simulink model "EV_assigment2"  (R2022a)
settings: Solver=VariableStepAuto  StartTime=0.0  StopTime=10800  RelTol=1e-3
libraries: spsCurrentMeasurementLib x141, spsSeriesRLCBranchLib x141, spsVoltageMeasurementLib x141, spsControlledVoltageSourceLib x140, spspowerguiLib x1
(part 8 of 15)

== system EV_assigment2/series/Subsystem15/Subsystem ==
  SOC : Inport
  Battery temp : Inport  Port=2
  2-D Lookup Table : Lookup_n-D  BreakpointsForDimension1=[0 0.10 0.20 0.30 0.40 0.50 0.60 0.70 0.80 0.90 1]  BreakpointsForDimension2=[293.15 313.15]  Table=[3.50 3.51;3.56 3.56; 3.60 3.62;3.64 3.66;3.67 3.69;3.71 3.72;3.79 3.81;3.88 3.89;3.97 3.99;4.08 4.08;4.19 4.19]  InternalRulePriority=Speed  RndMeth=Simplest
      settings: InputPortMap=u0,u1
  2-D Lookup Table1 : Lookup_n-D  BreakpointsForDimension1=[0 0.10 0.20 0.30 0.40 0.50 0.60 0.70 0.80 0.90 1]  BreakpointsForDimension2=[293.15 313.15]  Table=[0.011448 0.009001;0.011038 0.008966;0.011281 0.009126;0.011236 0.00911;0.010959 0.008957;0.010714 0.008797;0.010698 0.008913;0.010712 0.009052;0.010917 0.009044;0.011304 0.008899;0.01160 0.008902]  InternalRulePriority=Speed  RndMeth=Simplest
      settings: InputPortMap=u0,u1
  2-D Lookup Table2 : Lookup_n-D  BreakpointsForDimension1=[0 0.10 0.20 0.30 0.40 0.50 0.60 0.70 0.80 0.90 1]  BreakpointsForDimension2=[293.15 313.15]  Table=[0.010342 0;0.006732 0.10;0.005116 0.20;0.004345 0.30;0.003883 0.40;0.003423 0.50;0.003346 0.60;0.003322 0.70;0.00332 0.80;0.003289 0.90;0.002811 1]  InternalRulePriority=Speed  RndMeth=Simplest
      settings: InputPortMap=u0,u1
  2-D Lookup Table3 : Lookup_n-D  BreakpointsForDimension1=[0 0.10 0.20 0.30 0.40 0.50 0.60 0.70 0.8 0.9 1]  BreakpointsForDimension2=[293.15 313.15]  Table=[2287.7 11897;6122 24515;18460 42098;20975 44453;15254 33098;10440 24492;13903 32975;16694 40007;15784 35937;12165 26430;9118 24795]  InternalRulePriority=Speed  RndMeth=Simplest
      settings: InputPortMap=u0,u1
  Em : Outport
  R0 : Outport  Port=2
  R1 : Outport  Port=3
  C1 : Outport  Port=4
  wires:
  Battery temp/1 -> 2-D Lookup Table3/2, 2-D Lookup Table2/2, 2-D Lookup Table1/2, 2-D Lookup Table/2
  2-D Lookup Table3/1 -> C1/1
  2-D Lookup Table/1 -> Em/1
  SOC/1 -> 2-D Lookup Table3/1, 2-D Lookup Table2/1, 2-D Lookup Table1/1, 2-D Lookup Table/1
  2-D Lookup Table2/1 -> R1/1
  2-D Lookup Table1/1 -> R0/1

== system EV_assigment2/series/Subsystem15/Subsystem1 ==
  Battery Current : Inport
  InitCap(Ah) : Inport  Port=2
  Temp(K) : Inport  Port=3
  Capacity : Lookup_n-D  NumberOfTableDimensions=1  BreakpointsForDimension1=[283.15 313.15]  Table=[28 28]  InternalRulePriority=Speed  RndMeth=Simplest
  Charge accumilator : Integrator  InitialConditionSource=external  UpperSaturationLimit=1  LowerSaturationLimit=0
  Convert to Ah : Gain  Gain=-1/3600
  Divide : Product  Inputs=*/
  LoadAh : Outport
  SOC : Outport  Port=2
  wires:
  Charge accumilator/1 -> Divide/1, LoadAh/1
  Divide/1 -> SOC/1
  Temp(K)/1 -> Capacity/1
  Capacity/1 -> Divide/2
  Battery Current/1 -> Convert to Ah/1
  Convert to Ah/1 -> Charge accumilator/1
  InitCap(Ah)/1 -> Charge accumilator/2

== system EV_assigment2/series/Subsystem16/Subsystem ==
  SOC : Inport
  Battery temp : Inport  Port=2
  2-D Lookup Table : Lookup_n-D  BreakpointsForDimension1=[0 0.10 0.20 0.30 0.40 0.50 0.60 0.70 0.80 0.90 1]  BreakpointsForDimension2=[293.15 313.15]  Table=[3.50 3.51;3.56 3.56; 3.60 3.62;3.64 3.66;3.67 3.69;3.71 3.72;3.79 3.81;3.88 3.89;3.97 3.99;4.08 4.08;4.19 4.19]  InternalRulePriority=Speed  RndMeth=Simplest
      settings: InputPortMap=u0,u1
  2-D Lookup Table1 : Lookup_n-D  BreakpointsForDimension1=[0 0.10 0.20 0.30 0.40 0.50 0.60 0.70 0.80 0.90 1]  BreakpointsForDimension2=[293.15 313.15]  Table=[0.011448 0.009001;0.011038 0.008966;0.011281 0.009126;0.011236 0.00911;0.010959 0.008957;0.010714 0.008797;0.010698 0.008913;0.010712 0.009052;0.010917 0.009044;0.011304 0.008899;0.01160 0.008902]  InternalRulePriority=Speed  RndMeth=Simplest
      settings: InputPortMap=u0,u1
  2-D Lookup Table2 : Lookup_n-D  BreakpointsForDimension1=[0 0.10 0.20 0.30 0.40 0.50 0.60 0.70 0.80 0.90 1]  BreakpointsForDimension2=[293.15 313.15]  Table=[0.010342 0;0.006732 0.10;0.005116 0.20;0.004345 0.30;0.003883 0.40;0.003423 0.50;0.003346 0.60;0.003322 0.70;0.00332 0.80;0.003289 0.90;0.002811 1]  InternalRulePriority=Speed  RndMeth=Simplest
      settings: InputPortMap=u0,u1
  2-D Lookup Table3 : Lookup_n-D  BreakpointsForDimension1=[0 0.10 0.20 0.30 0.40 0.50 0.60 0.70 0.8 0.9 1]  BreakpointsForDimension2=[293.15 313.15]  Table=[2287.7 11897;6122 24515;18460 42098;20975 44453;15254 33098;10440 24492;13903 32975;16694 40007;15784 35937;12165 26430;9118 24795]  InternalRulePriority=Speed  RndMeth=Simplest
      settings: InputPortMap=u0,u1
  Em : Outport
  R0 : Outport  Port=2
  R1 : Outport  Port=3
  C1 : Outport  Port=4
  wires:
  Battery temp/1 -> 2-D Lookup Table3/2, 2-D Lookup Table2/2, 2-D Lookup Table1/2, 2-D Lookup Table/2
  2-D Lookup Table3/1 -> C1/1
  2-D Lookup Table/1 -> Em/1
  SOC/1 -> 2-D Lookup Table3/1, 2-D Lookup Table2/1, 2-D Lookup Table1/1, 2-D Lookup Table/1
  2-D Lookup Table2/1 -> R1/1
  2-D Lookup Table1/1 -> R0/1

== system EV_assigment2/series/Subsystem16/Subsystem1 ==
  Battery Current : Inport
  InitCap(Ah) : Inport  Port=2
  Temp(K) : Inport  Port=3
  Capacity : Lookup_n-D  NumberOfTableDimensions=1  BreakpointsForDimension1=[283.15 313.15]  Table=[28 28]  InternalRulePriority=Speed  RndMeth=Simplest
  Charge accumilator : Integrator  InitialConditionSource=external  UpperSaturationLimit=1  LowerSaturationLimit=0
  Convert to Ah : Gain  Gain=-1/3600
  Divide : Product  Inputs=*/
  LoadAh : Outport
  SOC : Outport  Port=2
  wires:
  Charge accumilator/1 -> Divide/1, LoadAh/1
  Divide/1 -> SOC/1
  Temp(K)/1 -> Capacity/1
  Capacity/1 -> Divide/2
  Battery Current/1 -> Convert to Ah/1
  Convert to Ah/1 -> Charge accumilator/1
  InitCap(Ah)/1 -> Charge accumilator/2

== system EV_assigment2/series/Subsystem17/Subsystem ==
  SOC : Inport
  Battery temp : Inport  Port=2
  2-D Lookup Table : Lookup_n-D  BreakpointsForDimension1=[0 0.10 0.20 0.30 0.40 0.50 0.60 0.70 0.80 0.90 1]  BreakpointsForDimension2=[293.15 313.15]  Table=[3.50 3.51;3.56 3.56; 3.60 3.62;3.64 3.66;3.67 3.69;3.71 3.72;3.79 3.81;3.88 3.89;3.97 3.99;4.08 4.08;4.19 4.19]  InternalRulePriority=Speed  RndMeth=Simplest
      settings: InputPortMap=u0,u1
  2-D Lookup Table1 : Lookup_n-D  BreakpointsForDimension1=[0 0.10 0.20 0.30 0.40 0.50 0.60 0.70 0.80 0.90 1]  BreakpointsForDimension2=[293.15 313.15]  Table=[0.011448 0.009001;0.011038 0.008966;0.011281 0.009126;0.011236 0.00911;0.010959 0.008957;0.010714 0.008797;0.010698 0.008913;0.010712 0.009052;0.010917 0.009044;0.011304 0.008899;0.01160 0.008902]  InternalRulePriority=Speed  RndMeth=Simplest
      settings: InputPortMap=u0,u1
  2-D Lookup Table2 : Lookup_n-D  BreakpointsForDimension1=[0 0.10 0.20 0.30 0.40 0.50 0.60 0.70 0.80 0.90 1]  BreakpointsForDimension2=[293.15 313.15]  Table=[0.010342 0;0.006732 0.10;0.005116 0.20;0.004345 0.30;0.003883 0.40;0.003423 0.50;0.003346 0.60;0.003322 0.70;0.00332 0.80;0.003289 0.90;0.002811 1]  InternalRulePriority=Speed  RndMeth=Simplest
      settings: InputPortMap=u0,u1
  2-D Lookup Table3 : Lookup_n-D  BreakpointsForDimension1=[0 0.10 0.20 0.30 0.40 0.50 0.60 0.70 0.8 0.9 1]  BreakpointsForDimension2=[293.15 313.15]  Table=[2287.7 11897;6122 24515;18460 42098;20975 44453;15254 33098;10440 24492;13903 32975;16694 40007;15784 35937;12165 26430;9118 24795]  InternalRulePriority=Speed  RndMeth=Simplest
      settings: InputPortMap=u0,u1
  Em : Outport
  R0 : Outport  Port=2
  R1 : Outport  Port=3
  C1 : Outport  Port=4
  wires:
  Battery temp/1 -> 2-D Lookup Table3/2, 2-D Lookup Table2/2, 2-D Lookup Table1/2, 2-D Lookup Table/2
  2-D Lookup Table3/1 -> C1/1
  2-D Lookup Table/1 -> Em/1
  SOC/1 -> 2-D Lookup Table3/1, 2-D Lookup Table2/1, 2-D Lookup Table1/1, 2-D Lookup Table/1
  2-D Lookup Table2/1 -> R1/1
  2-D Lookup Table1/1 -> R0/1

== system EV_assigment2/series/Subsystem17/Subsystem1 ==
  Battery Current : Inport
  InitCap(Ah) : Inport  Port=2
  Temp(K) : Inport  Port=3
  Capacity : Lookup_n-D  NumberOfTableDimensions=1  BreakpointsForDimension1=[283.15 313.15]  Table=[28 28]  InternalRulePriority=Speed  RndMeth=Simplest
  Charge accumilator : Integrator  InitialConditionSource=external  UpperSaturationLimit=1  LowerSaturationLimit=0
  Convert to Ah : Gain  Gain=-1/3600
  Divide : Product  Inputs=*/
  LoadAh : Outport
  SOC : Outport  Port=2
  wires:
  Charge accumilator/1 -> Divide/1, LoadAh/1
  Divide/1 -> SOC/1
  Temp(K)/1 -> Capacity/1
  Capacity/1 -> Divide/2
  Battery Current/1 -> Convert to Ah/1
  Convert to Ah/1 -> Charge accumilator/1
  InitCap(Ah)/1 -> Charge accumilator/2

== system EV_assigment2/series/Subsystem18/Subsystem ==
  SOC : Inport
  Battery temp : Inport  Port=2
  2-D Lookup Table : Lookup_n-D  BreakpointsForDimension1=[0 0.10 0.20 0.30 0.40 0.50 0.60 0.70 0.80 0.90 1]  BreakpointsForDimension2=[293.15 313.15]  Table=[3.50 3.51;3.56 3.56; 3.60 3.62;3.64 3.66;3.67 3.69;3.71 3.72;3.79 3.81;3.88 3.89;3.97 3.99;4.08 4.08;4.19 4.19]  InternalRulePriority=Speed  RndMeth=Simplest
      settings: InputPortMap=u0,u1
  2-D Lookup Table1 : Lookup_n-D  BreakpointsForDimension1=[0 0.10 0.20 0.30 0.40 0.50 0.60 0.70 0.80 0.90 1]  BreakpointsForDimension2=[293.15 313.15]  Table=[0.011448 0.009001;0.011038 0.008966;0.011281 0.009126;0.011236 0.00911;0.010959 0.008957;0.010714 0.008797;0.010698 0.008913;0.010712 0.009052;0.010917 0.009044;0.011304 0.008899;0.01160 0.008902]  InternalRulePriority=Speed  RndMeth=Simplest
      settings: InputPortMap=u0,u1
  2-D Lookup Table2 : Lookup_n-D  BreakpointsForDimension1=[0 0.10 0.20 0.30 0.40 0.50 0.60 0.70 0.80 0.90 1]  BreakpointsForDimension2=[293.15 313.15]  Table=[0.010342 0;0.006732 0.10;0.005116 0.20;0.004345 0.30;0.003883 0.40;0.003423 0.50;0.003346 0.60;0.003322 0.70;0.00332 0.80;0.003289 0.90;0.002811 1]  InternalRulePriority=Speed  RndMeth=Simplest
      settings: InputPortMap=u0,u1
  2-D Lookup Table3 : Lookup_n-D  BreakpointsForDimension1=[0 0.10 0.20 0.30 0.40 0.50 0.60 0.70 0.8 0.9 1]  BreakpointsForDimension2=[293.15 313.15]  Table=[2287.7 11897;6122 24515;18460 42098;20975 44453;15254 33098;10440 24492;13903 32975;16694 40007;15784 35937;12165 26430;9118 24795]  InternalRulePriority=Speed  RndMeth=Simplest
      settings: InputPortMap=u0,u1
  Em : Outport
  R0 : Outport  Port=2
  R1 : Outport  Port=3
  C1 : Outport  Port=4
  wires:
  Battery temp/1 -> 2-D Lookup Table3/2, 2-D Lookup Table2/2, 2-D Lookup Table1/2, 2-D Lookup Table/2
  2-D Lookup Table3/1 -> C1/1
  2-D Lookup Table/1 -> Em/1
  SOC/1 -> 2-D Lookup Table3/1, 2-D Lookup Table2/1, 2-D Lookup Table1/1, 2-D Lookup Table/1
  2-D Lookup Table2/1 -> R1/1
  2-D Lookup Table1/1 -> R0/1

== system EV_assigment2/series/Subsystem18/Subsystem1 ==
  Battery Current : Inport
  InitCap(Ah) : Inport  Port=2
  Temp(K) : Inport  Port=3
  Capacity : Lookup_n-D  NumberOfTableDimensions=1  BreakpointsForDimension1=[283.15 313.15]  Table=[28 28]  InternalRulePriority=Speed  RndMeth=Simplest
  Charge accumilator : Integrator  InitialConditionSource=external  UpperSaturationLimit=1  LowerSaturationLimit=0
  Convert to Ah : Gain  Gain=-1/3600
  Divide : Product  Inputs=*/
  LoadAh : Outport
  SOC : Outport  Port=2
  wires:
  Charge accumilator/1 -> Divide/1, LoadAh/1
  Divide/1 -> SOC/1
  Temp(K)/1 -> Capacity/1
  Capacity/1 -> Divide/2
  Battery Current/1 -> Convert to Ah/1
  Convert to Ah/1 -> Charge accumilator/1
  InitCap(Ah)/1 -> Charge accumilator/2

== system EV_assigment2/series/Subsystem19/Subsystem ==
  SOC : Inport
  Battery temp : Inport  Port=2
  2-D Lookup Table : Lookup_n-D  BreakpointsForDimension1=[0 0.10 0.20 0.30 0.40 0.50 0.60 0.70 0.80 0.90 1]  BreakpointsForDimension2=[293.15 313.15]  Table=[3.50 3.51;3.56 3.56; 3.60 3.62;3.64 3.66;3.67 3.69;3.71 3.72;3.79 3.81;3.88 3.89;3.97 3.99;4.08 4.08;4.19 4.19]  InternalRulePriority=Speed  RndMeth=Simplest
      settings: InputPortMap=u0,u1
  2-D Lookup Table1 : Lookup_n-D  BreakpointsForDimension1=[0 0.10 0.20 0.30 0.40 0.50 0.60 0.70 0.80 0.90 1]  BreakpointsForDimension2=[293.15 313.15]  Table=[0.011448 0.009001;0.011038 0.008966;0.011281 0.009126;0.011236 0.00911;0.010959 0.008957;0.010714 0.008797;0.010698 0.008913;0.010712 0.009052;0.010917 0.009044;0.011304 0.008899;0.01160 0.008902]  InternalRulePriority=Speed  RndMeth=Simplest
      settings: InputPortMap=u0,u1
  2-D Lookup Table2 : Lookup_n-D  BreakpointsForDimension1=[0 0.10 0.20 0.30 0.40 0.50 0.60 0.70 0.80 0.90 1]  BreakpointsForDimension2=[293.15 313.15]  Table=[0.010342 0;0.006732 0.10;0.005116 0.20;0.004345 0.30;0.003883 0.40;0.003423 0.50;0.003346 0.60;0.003322 0.70;0.00332 0.80;0.003289 0.90;0.002811 1]  InternalRulePriority=Speed  RndMeth=Simplest
      settings: InputPortMap=u0,u1
  2-D Lookup Table3 : Lookup_n-D  BreakpointsForDimension1=[0 0.10 0.20 0.30 0.40 0.50 0.60 0.70 0.8 0.9 1]  BreakpointsForDimension2=[293.15 313.15]  Table=[2287.7 11897;6122 24515;18460 42098;20975 44453;15254 33098;10440 24492;13903 32975;16694 40007;15784 35937;12165 26430;9118 24795]  InternalRulePriority=Speed  RndMeth=Simplest
      settings: InputPortMap=u0,u1
  Em : Outport
  R0 : Outport  Port=2
  R1 : Outport  Port=3
  C1 : Outport  Port=4
  wires:
  Battery temp/1 -> 2-D Lookup Table3/2, 2-D Lookup Table2/2, 2-D Lookup Table1/2, 2-D Lookup Table/2
  2-D Lookup Table3/1 -> C1/1
  2-D Lookup Table/1 -> Em/1
  SOC/1 -> 2-D Lookup Table3/1, 2-D Lookup Table2/1, 2-D Lookup Table1/1, 2-D Lookup Table/1
  2-D Lookup Table2/1 -> R1/1
  2-D Lookup Table1/1 -> R0/1

== system EV_assigment2/series/Subsystem19/Subsystem1 ==
  Battery Current : Inport
  InitCap(Ah) : Inport  Port=2
  Temp(K) : Inport  Port=3
  Capacity : Lookup_n-D  NumberOfTableDimensions=1  BreakpointsForDimension1=[283.15 313.15]  Table=[28 28]  InternalRulePriority=Speed  RndMeth=Simplest
  Charge accumilator : Integrator  InitialConditionSource=external  UpperSaturationLimit=1  LowerSaturationLimit=0
  Convert to Ah : Gain  Gain=-1/3600
  Divide : Product  Inputs=*/
  LoadAh : Outport
  SOC : Outport  Port=2
  wires:
  Charge accumilator/1 -> Divide/1, LoadAh/1
  Divide/1 -> SOC/1
  Temp(K)/1 -> Capacity/1
  Capacity/1 -> Divide/2
  Battery Current/1 -> Convert to Ah/1
  Convert to Ah/1 -> Charge accumilator/1
  InitCap(Ah)/1 -> Charge accumilator/2

== system EV_assigment2/series/Subsystem2/Subsystem ==
  SOC : Inport
  Battery temp : Inport  Port=2
  2-D Lookup Table : Lookup_n-D  BreakpointsForDimension1=[0 0.10 0.20 0.30 0.40 0.50 0.60 0.70 0.80 0.90 1]  BreakpointsForDimension2=[293.15 313.15]  Table=[3.50 3.51;3.56 3.56; 3.60 3.62;3.64 3.66;3.67 3.69;3.71 3.72;3.79 3.81;3.88 3.89;3.97 3.99;4.08 4.08;4.19 4.19]  InternalRulePriority=Speed  RndMeth=Simplest
      settings: InputPortMap=u0,u1
  2-D Lookup Table1 : Lookup_n-D  BreakpointsForDimension1=[0 0.10 0.20 0.30 0.40 0.50 0.60 0.70 0.80 0.90 1]  BreakpointsForDimension2=[293.15 313.15]  Table=[0.011448 0.009001;0.011038 0.008966;0.011281 0.009126;0.011236 0.00911;0.010959 0.008957;0.010714 0.008797;0.010698 0.008913;0.010712 0.009052;0.010917 0.009044;0.011304 0.008899;0.01160 0.008902]  InternalRulePriority=Speed  RndMeth=Simplest
      settings: InputPortMap=u0,u1
  2-D Lookup Table2 : Lookup_n-D  BreakpointsForDimension1=[0 0.10 0.20 0.30 0.40 0.50 0.60 0.70 0.80 0.90 1]  BreakpointsForDimension2=[293.15 313.15]  Table=[0.010342 0;0.006732 0.10;0.005116 0.20;0.004345 0.30;0.003883 0.40;0.003423 0.50;0.003346 0.60;0.003322 0.70;0.00332 0.80;0.003289 0.90;0.002811 1]  InternalRulePriority=Speed  RndMeth=Simplest
      settings: InputPortMap=u0,u1
  2-D Lookup Table3 : Lookup_n-D  BreakpointsForDimension1=[0 0.10 0.20 0.30 0.40 0.50 0.60 0.70 0.8 0.9 1]  BreakpointsForDimension2=[293.15 313.15]  Table=[2287.7 11897;6122 24515;18460 42098;20975 44453;15254 33098;10440 24492;13903 32975;16694 40007;15784 35937;12165 26430;9118 24795]  InternalRulePriority=Speed  RndMeth=Simplest
      settings: InputPortMap=u0,u1
  Em : Outport
  R0 : Outport  Port=2
  R1 : Outport  Port=3
  C1 : Outport  Port=4
  wires:
  Battery temp/1 -> 2-D Lookup Table3/2, 2-D Lookup Table2/2, 2-D Lookup Table1/2, 2-D Lookup Table/2
  2-D Lookup Table3/1 -> C1/1
  2-D Lookup Table/1 -> Em/1
  SOC/1 -> 2-D Lookup Table3/1, 2-D Lookup Table2/1, 2-D Lookup Table1/1, 2-D Lookup Table/1
  2-D Lookup Table2/1 -> R1/1
  2-D Lookup Table1/1 -> R0/1

== system EV_assigment2/series/Subsystem2/Subsystem1 ==
  Battery Current : Inport
  InitCap(Ah) : Inport  Port=2
  Temp(K) : Inport  Port=3
  Capacity : Lookup_n-D  NumberOfTableDimensions=1  BreakpointsForDimension1=[283.15 313.15]  Table=[28 28]  InternalRulePriority=Speed  RndMeth=Simplest
  Charge accumilator : Integrator  InitialConditionSource=external  UpperSaturationLimit=1  LowerSaturationLimit=0
  Convert to Ah : Gain  Gain=-1/3600
  Divide : Product  Inputs=*/
  LoadAh : Outport
  SOC : Outport  Port=2
  wires:
  Charge accumilator/1 -> Divide/1, LoadAh/1
  Divide/1 -> SOC/1
  Temp(K)/1 -> Capacity/1
  Capacity/1 -> Divide/2
  Battery Current/1 -> Convert to Ah/1
  Convert to Ah/1 -> Charge accumilator/1
  InitCap(Ah)/1 -> Charge accumilator/2

== system EV_assigment2/series/Subsystem20/Subsystem ==
  SOC : Inport
  Battery temp : Inport  Port=2
  2-D Lookup Table : Lookup_n-D  BreakpointsForDimension1=[0 0.10 0.20 0.30 0.40 0.50 0.60 0.70 0.80 0.90 1]  BreakpointsForDimension2=[293.15 313.15]  Table=[3.50 3.51;3.56 3.56; 3.60 3.62;3.64 3.66;3.67 3.69;3.71 3.72;3.79 3.81;3.88 3.89;3.97 3.99;4.08 4.08;4.19 4.19]  InternalRulePriority=Speed  RndMeth=Simplest
      settings: InputPortMap=u0,u1
  2-D Lookup Table1 : Lookup_n-D  BreakpointsForDimension1=[0 0.10 0.20 0.30 0.40 0.50 0.60 0.70 0.80 0.90 1]  BreakpointsForDimension2=[293.15 313.15]  Table=[0.011448 0.009001;0.011038 0.008966;0.011281 0.009126;0.011236 0.00911;0.010959 0.008957;0.010714 0.008797;0.010698 0.008913;0.010712 0.009052;0.010917 0.009044;0.011304 0.008899;0.01160 0.008902]  InternalRulePriority=Speed  RndMeth=Simplest
      settings: InputPortMap=u0,u1
  2-D Lookup Table2 : Lookup_n-D  BreakpointsForDimension1=[0 0.10 0.20 0.30 0.40 0.50 0.60 0.70 0.80 0.90 1]  BreakpointsForDimension2=[293.15 313.15]  Table=[0.010342 0;0.006732 0.10;0.005116 0.20;0.004345 0.30;0.003883 0.40;0.003423 0.50;0.003346 0.60;0.003322 0.70;0.00332 0.80;0.003289 0.90;0.002811 1]  InternalRulePriority=Speed  RndMeth=Simplest
      settings: InputPortMap=u0,u1
  2-D Lookup Table3 : Lookup_n-D  BreakpointsForDimension1=[0 0.10 0.20 0.30 0.40 0.50 0.60 0.70 0.8 0.9 1]  BreakpointsForDimension2=[293.15 313.15]  Table=[2287.7 11897;6122 24515;18460 42098;20975 44453;15254 33098;10440 24492;13903 32975;16694 40007;15784 35937;12165 26430;9118 24795]  InternalRulePriority=Speed  RndMeth=Simplest
      settings: InputPortMap=u0,u1
  Em : Outport
  R0 : Outport  Port=2
  R1 : Outport  Port=3
  C1 : Outport  Port=4
  wires:
  Battery temp/1 -> 2-D Lookup Table3/2, 2-D Lookup Table2/2, 2-D Lookup Table1/2, 2-D Lookup Table/2
  2-D Lookup Table3/1 -> C1/1
  2-D Lookup Table/1 -> Em/1
  SOC/1 -> 2-D Lookup Table3/1, 2-D Lookup Table2/1, 2-D Lookup Table1/1, 2-D Lookup Table/1
  2-D Lookup Table2/1 -> R1/1
  2-D Lookup Table1/1 -> R0/1

== system EV_assigment2/series/Subsystem20/Subsystem1 ==
  Battery Current : Inport
  InitCap(Ah) : Inport  Port=2
  Temp(K) : Inport  Port=3
  Capacity : Lookup_n-D  NumberOfTableDimensions=1  BreakpointsForDimension1=[283.15 313.15]  Table=[28 28]  InternalRulePriority=Speed  RndMeth=Simplest
  Charge accumilator : Integrator  InitialConditionSource=external  UpperSaturationLimit=1  LowerSaturationLimit=0
  Convert to Ah : Gain  Gain=-1/3600
  Divide : Product  Inputs=*/
  LoadAh : Outport
  SOC : Outport  Port=2
  wires:
  Charge accumilator/1 -> Divide/1, LoadAh/1
  Divide/1 -> SOC/1
  Temp(K)/1 -> Capacity/1
  Capacity/1 -> Divide/2
  Battery Current/1 -> Convert to Ah/1
  Convert to Ah/1 -> Charge accumilator/1
  InitCap(Ah)/1 -> Charge accumilator/2

== system EV_assigment2/series/Subsystem21/Subsystem ==
  SOC : Inport
  Battery temp : Inport  Port=2
  2-D Lookup Table : Lookup_n-D  BreakpointsForDimension1=[0 0.10 0.20 0.30 0.40 0.50 0.60 0.70 0.80 0.90 1]  BreakpointsForDimension2=[293.15 313.15]  Table=[3.50 3.51;3.56 3.56; 3.60 3.62;3.64 3.66;3.67 3.69;3.71 3.72;3.79 3.81;3.88 3.89;3.97 3.99;4.08 4.08;4.19 4.19]  InternalRulePriority=Speed  RndMeth=Simplest
      settings: InputPortMap=u0,u1
  2-D Lookup Table1 : Lookup_n-D  BreakpointsForDimension1=[0 0.10 0.20 0.30 0.40 0.50 0.60 0.70 0.80 0.90 1]  BreakpointsForDimension2=[293.15 313.15]  Table=[0.011448 0.009001;0.011038 0.008966;0.011281 0.009126;0.011236 0.00911;0.010959 0.008957;0.010714 0.008797;0.010698 0.008913;0.010712 0.009052;0.010917 0.009044;0.011304 0.008899;0.01160 0.008902]  InternalRulePriority=Speed  RndMeth=Simplest
      settings: InputPortMap=u0,u1
  2-D Lookup Table2 : Lookup_n-D  BreakpointsForDimension1=[0 0.10 0.20 0.30 0.40 0.50 0.60 0.70 0.80 0.90 1]  BreakpointsForDimension2=[293.15 313.15]  Table=[0.010342 0;0.006732 0.10;0.005116 0.20;0.004345 0.30;0.003883 0.40;0.003423 0.50;0.003346 0.60;0.003322 0.70;0.00332 0.80;0.003289 0.90;0.002811 1]  InternalRulePriority=Speed  RndMeth=Simplest
      settings: InputPortMap=u0,u1
  2-D Lookup Table3 : Lookup_n-D  BreakpointsForDimension1=[0 0.10 0.20 0.30 0.40 0.50 0.60 0.70 0.8 0.9 1]  BreakpointsForDimension2=[293.15 313.15]  Table=[2287.7 11897;6122 24515;18460 42098;20975 44453;15254 33098;10440 24492;13903 32975;16694 40007;15784 35937;12165 26430;9118 24795]  InternalRulePriority=Speed  RndMeth=Simplest
      settings: InputPortMap=u0,u1
  Em : Outport
  R0 : Outport  Port=2
  R1 : Outport  Port=3
  C1 : Outport  Port=4
  wires:
  Battery temp/1 -> 2-D Lookup Table3/2, 2-D Lookup Table2/2, 2-D Lookup Table1/2, 2-D Lookup Table/2
  2-D Lookup Table3/1 -> C1/1
  2-D Lookup Table/1 -> Em/1
  SOC/1 -> 2-D Lookup Table3/1, 2-D Lookup Table2/1, 2-D Lookup Table1/1, 2-D Lookup Table/1
  2-D Lookup Table2/1 -> R1/1
  2-D Lookup Table1/1 -> R0/1

== system EV_assigment2/series/Subsystem21/Subsystem1 ==
  Battery Current : Inport
  InitCap(Ah) : Inport  Port=2
  Temp(K) : Inport  Port=3
  Capacity : Lookup_n-D  NumberOfTableDimensions=1  BreakpointsForDimension1=[283.15 313.15]  Table=[28 28]  InternalRulePriority=Speed  RndMeth=Simplest
  Charge accumilator : Integrator  InitialConditionSource=external  UpperSaturationLimit=1  LowerSaturationLimit=0
  Convert to Ah : Gain  Gain=-1/3600
  Divide : Product  Inputs=*/
  LoadAh : Outport
  SOC : Outport  Port=2
  wires:
  Charge accumilator/1 -> Divide/1, LoadAh/1
  Divide/1 -> SOC/1
  Temp(K)/1 -> Capacity/1
  Capacity/1 -> Divide/2
  Battery Current/1 -> Convert to Ah/1
  Convert to Ah/1 -> Charge accumilator/1
  InitCap(Ah)/1 -> Charge accumilator/2

== system EV_assigment2/series/Subsystem22/Subsystem ==
  SOC : Inport
  Battery temp : Inport  Port=2
  2-D Lookup Table : Lookup_n-D  BreakpointsForDimension1=[0 0.10 0.20 0.30 0.40 0.50 0.60 0.70 0.80 0.90 1]  BreakpointsForDimension2=[293.15 313.15]  Table=[3.50 3.51;3.56 3.56; 3.60 3.62;3.64 3.66;3.67 3.69;3.71 3.72;3.79 3.81;3.88 3.89;3.97 3.99;4.08 4.08;4.19 4.19]  InternalRulePriority=Speed  RndMeth=Simplest
      settings: InputPortMap=u0,u1
  2-D Lookup Table1 : Lookup_n-D  BreakpointsForDimension1=[0 0.10 0.20 0.30 0.40 0.50 0.60 0.70 0.80 0.90 1]  BreakpointsForDimension2=[293.15 313.15]  Table=[0.011448 0.009001;0.011038 0.008966;0.011281 0.009126;0.011236 0.00911;0.010959 0.008957;0.010714 0.008797;0.010698 0.008913;0.010712 0.009052;0.010917 0.009044;0.011304 0.008899;0.01160 0.008902]  InternalRulePriority=Speed  RndMeth=Simplest
      settings: InputPortMap=u0,u1
  2-D Lookup Table2 : Lookup_n-D  BreakpointsForDimension1=[0 0.10 0.20 0.30 0.40 0.50 0.60 0.70 0.80 0.90 1]  BreakpointsForDimension2=[293.15 313.15]  Table=[0.010342 0;0.006732 0.10;0.005116 0.20;0.004345 0.30;0.003883 0.40;0.003423 0.50;0.003346 0.60;0.003322 0.70;0.00332 0.80;0.003289 0.90;0.002811 1]  InternalRulePriority=Speed  RndMeth=Simplest
      settings: InputPortMap=u0,u1
  2-D Lookup Table3 : Lookup_n-D  BreakpointsForDimension1=[0 0.10 0.20 0.30 0.40 0.50 0.60 0.70 0.8 0.9 1]  BreakpointsForDimension2=[293.15 313.15]  Table=[2287.7 11897;6122 24515;18460 42098;20975 44453;15254 33098;10440 24492;13903 32975;16694 40007;15784 35937;12165 26430;9118 24795]  InternalRulePriority=Speed  RndMeth=Simplest
      settings: InputPortMap=u0,u1
  Em : Outport
  R0 : Outport  Port=2
  R1 : Outport  Port=3
  C1 : Outport  Port=4
  wires:
  Battery temp/1 -> 2-D Lookup Table3/2, 2-D Lookup Table2/2, 2-D Lookup Table1/2, 2-D Lookup Table/2
  2-D Lookup Table3/1 -> C1/1
  2-D Lookup Table/1 -> Em/1
  SOC/1 -> 2-D Lookup Table3/1, 2-D Lookup Table2/1, 2-D Lookup Table1/1, 2-D Lookup Table/1
  2-D Lookup Table2/1 -> R1/1
  2-D Lookup Table1/1 -> R0/1

== system EV_assigment2/series/Subsystem22/Subsystem1 ==
  Battery Current : Inport
  InitCap(Ah) : Inport  Port=2
  Temp(K) : Inport  Port=3
  Capacity : Lookup_n-D  NumberOfTableDimensions=1  BreakpointsForDimension1=[283.15 313.15]  Table=[28 28]  InternalRulePriority=Speed  RndMeth=Simplest
  Charge accumilator : Integrator  InitialConditionSource=external  UpperSaturationLimit=1  LowerSaturationLimit=0
  Convert to Ah : Gain  Gain=-1/3600
  Divide : Product  Inputs=*/
  LoadAh : Outport
  SOC : Outport  Port=2
  wires:
  Charge accumilator/1 -> Divide/1, LoadAh/1
  Divide/1 -> SOC/1
  Temp(K)/1 -> Capacity/1
  Capacity/1 -> Divide/2
  Battery Current/1 -> Convert to Ah/1
  Convert to Ah/1 -> Charge accumilator/1
  InitCap(Ah)/1 -> Charge accumilator/2

== system EV_assigment2/series/Subsystem23/Subsystem ==
  SOC : Inport
  Battery temp : Inport  Port=2
  2-D Lookup Table : Lookup_n-D  BreakpointsForDimension1=[0 0.10 0.20 0.30 0.40 0.50 0.60 0.70 0.80 0.90 1]  BreakpointsForDimension2=[293.15 313.15]  Table=[3.50 3.51;3.56 3.56; 3.60 3.62;3.64 3.66;3.67 3.69;3.71 3.72;3.79 3.81;3.88 3.89;3.97 3.99;4.08 4.08;4.19 4.19]  InternalRulePriority=Speed  RndMeth=Simplest
      settings: InputPortMap=u0,u1
  2-D Lookup Table1 : Lookup_n-D  BreakpointsForDimension1=[0 0.10 0.20 0.30 0.40 0.50 0.60 0.70 0.80 0.90 1]  BreakpointsForDimension2=[293.15 313.15]  Table=[0.011448 0.009001;0.011038 0.008966;0.011281 0.009126;0.011236 0.00911;0.010959 0.008957;0.010714 0.008797;0.010698 0.008913;0.010712 0.009052;0.010917 0.009044;0.011304 0.008899;0.01160 0.008902]  InternalRulePriority=Speed  RndMeth=Simplest
      settings: InputPortMap=u0,u1
  2-D Lookup Table2 : Lookup_n-D  BreakpointsForDimension1=[0 0.10 0.20 0.30 0.40 0.50 0.60 0.70 0.80 0.90 1]  BreakpointsForDimension2=[293.15 313.15]  Table=[0.010342 0;0.006732 0.10;0.005116 0.20;0.004345 0.30;0.003883 0.40;0.003423 0.50;0.003346 0.60;0.003322 0.70;0.00332 0.80;0.003289 0.90;0.002811 1]  InternalRulePriority=Speed  RndMeth=Simplest
      settings: InputPortMap=u0,u1
  2-D Lookup Table3 : Lookup_n-D  BreakpointsForDimension1=[0 0.10 0.20 0.30 0.40 0.50 0.60 0.70 0.8 0.9 1]  BreakpointsForDimension2=[293.15 313.15]  Table=[2287.7 11897;6122 24515;18460 42098;20975 44453;15254 33098;10440 24492;13903 32975;16694 40007;15784 35937;12165 26430;9118 24795]  InternalRulePriority=Speed  RndMeth=Simplest
      settings: InputPortMap=u0,u1
  Em : Outport
  R0 : Outport  Port=2
  R1 : Outport  Port=3
  C1 : Outport  Port=4
  wires:
  Battery temp/1 -> 2-D Lookup Table3/2, 2-D Lookup Table2/2, 2-D Lookup Table1/2, 2-D Lookup Table/2
  2-D Lookup Table3/1 -> C1/1
  2-D Lookup Table/1 -> Em/1
  SOC/1 -> 2-D Lookup Table3/1, 2-D Lookup Table2/1, 2-D Lookup Table1/1, 2-D Lookup Table/1
  2-D Lookup Table2/1 -> R1/1
  2-D Lookup Table1/1 -> R0/1

== system EV_assigment2/series/Subsystem23/Subsystem1 ==
  Battery Current : Inport
  InitCap(Ah) : Inport  Port=2
  Temp(K) : Inport  Port=3
  Capacity : Lookup_n-D  NumberOfTableDimensions=1  BreakpointsForDimension1=[283.15 313.15]  Table=[28 28]  InternalRulePriority=Speed  RndMeth=Simplest
  Charge accumilator : Integrator  InitialConditionSource=external  UpperSaturationLimit=1  LowerSaturationLimit=0
  Convert to Ah : Gain  Gain=-1/3600
  Divide : Product  Inputs=*/
  LoadAh : Outport
  SOC : Outport  Port=2
  wires:
  Charge accumilator/1 -> Divide/1, LoadAh/1
  Divide/1 -> SOC/1
  Temp(K)/1 -> Capacity/1
  Capacity/1 -> Divide/2
  Battery Current/1 -> Convert to Ah/1
  Convert to Ah/1 -> Charge accumilator/1
  InitCap(Ah)/1 -> Charge accumilator/2

== system EV_assigment2/series/Subsystem24/Subsystem ==
  SOC : Inport
  Battery temp : Inport  Port=2
  2-D Lookup Table : Lookup_n-D  BreakpointsForDimension1=[0 0.10 0.20 0.30 0.40 0.50 0.60 0.70 0.80 0.90 1]  BreakpointsForDimension2=[293.15 313.15]  Table=[3.50 3.51;3.56 3.56; 3.60 3.62;3.64 3.66;3.67 3.69;3.71 3.72;3.79 3.81;3.88 3.89;3.97 3.99;4.08 4.08;4.19 4.19]  InternalRulePriority=Speed  RndMeth=Simplest
      settings: InputPortMap=u0,u1
  2-D Lookup Table1 : Lookup_n-D  BreakpointsForDimension1=[0 0.10 0.20 0.30 0.40 0.50 0.60 0.70 0.80 0.90 1]  BreakpointsForDimension2=[293.15 313.15]  Table=[0.011448 0.009001;0.011038 0.008966;0.011281 0.009126;0.011236 0.00911;0.010959 0.008957;0.010714 0.008797;0.010698 0.008913;0.010712 0.009052;0.010917 0.009044;0.011304 0.008899;0.01160 0.008902]  InternalRulePriority=Speed  RndMeth=Simplest
      settings: InputPortMap=u0,u1
  2-D Lookup Table2 : Lookup_n-D  BreakpointsForDimension1=[0 0.10 0.20 0.30 0.40 0.50 0.60 0.70 0.80 0.90 1]  BreakpointsForDimension2=[293.15 313.15]  Table=[0.010342 0;0.006732 0.10;0.005116 0.20;0.004345 0.30;0.003883 0.40;0.003423 0.50;0.003346 0.60;0.003322 0.70;0.00332 0.80;0.003289 0.90;0.002811 1]  InternalRulePriority=Speed  RndMeth=Simplest
      settings: InputPortMap=u0,u1
  2-D Lookup Table3 : Lookup_n-D  BreakpointsForDimension1=[0 0.10 0.20 0.30 0.40 0.50 0.60 0.70 0.8 0.9 1]  BreakpointsForDimension2=[293.15 313.15]  Table=[2287.7 11897;6122 24515;18460 42098;20975 44453;15254 33098;10440 24492;13903 32975;16694 40007;15784 35937;12165 26430;9118 24795]  InternalRulePriority=Speed  RndMeth=Simplest
      settings: InputPortMap=u0,u1
  Em : Outport
  R0 : Outport  Port=2
  R1 : Outport  Port=3
  C1 : Outport  Port=4
  wires:
  Battery temp/1 -> 2-D Lookup Table3/2, 2-D Lookup Table2/2, 2-D Lookup Table1/2, 2-D Lookup Table/2
  2-D Lookup Table3/1 -> C1/1
  2-D Lookup Table/1 -> Em/1
  SOC/1 -> 2-D Lookup Table3/1, 2-D Lookup Table2/1, 2-D Lookup Table1/1, 2-D Lookup Table/1
  2-D Lookup Table2/1 -> R1/1
  2-D Lookup Table1/1 -> R0/1

== system EV_assigment2/series/Subsystem24/Subsystem1 ==
  Battery Current : Inport
  InitCap(Ah) : Inport  Port=2
  Temp(K) : Inport  Port=3
  Capacity : Lookup_n-D  NumberOfTableDimensions=1  BreakpointsForDimension1=[283.15 313.15]  Table=[28 28]  InternalRulePriority=Speed  RndMeth=Simplest
  Charge accumilator : Integrator  InitialConditionSource=external  UpperSaturationLimit=1  LowerSaturationLimit=0
  Convert to Ah : Gain  Gain=-1/3600
  Divide : Product  Inputs=*/
  LoadAh : Outport
  SOC : Outport  Port=2
  wires:
  Charge accumilator/1 -> Divide/1, LoadAh/1
  Divide/1 -> SOC/1
  Temp(K)/1 -> Capacity/1
  Capacity/1 -> Divide/2
  Battery Current/1 -> Convert to Ah/1
  Convert to Ah/1 -> Charge accumilator/1
  InitCap(Ah)/1 -> Charge accumilator/2

== system EV_assigment2/series/Subsystem25/Subsystem ==
  SOC : Inport
  Battery temp : Inport  Port=2
  2-D Lookup Table : Lookup_n-D  BreakpointsForDimension1=[0 0.10 0.20 0.30 0.40 0.50 0.60 0.70 0.80 0.90 1]  BreakpointsForDimension2=[293.15 313.15]  Table=[3.50 3.51;3.56 3.56; 3.60 3.62;3.64 3.66;3.67 3.69;3.71 3.72;3.79 3.81;3.88 3.89;3.97 3.99;4.08 4.08;4.19 4.19]  InternalRulePriority=Speed  RndMeth=Simplest
      settings: InputPortMap=u0,u1
  2-D Lookup Table1 : Lookup_n-D  BreakpointsForDimension1=[0 0.10 0.20 0.30 0.40 0.50 0.60 0.70 0.80 0.90 1]  BreakpointsForDimension2=[293.15 313.15]  Table=[0.011448 0.009001;0.011038 0.008966;0.011281 0.009126;0.011236 0.00911;0.010959 0.008957;0.010714 0.008797;0.010698 0.008913;0.010712 0.009052;0.010917 0.009044;0.011304 0.008899;0.01160 0.008902]  InternalRulePriority=Speed  RndMeth=Simplest
      settings: InputPortMap=u0,u1
  2-D Lookup Table2 : Lookup_n-D  BreakpointsForDimension1=[0 0.10 0.20 0.30 0.40 0.50 0.60 0.70 0.80 0.90 1]  BreakpointsForDimension2=[293.15 313.15]  Table=[0.010342 0;0.006732 0.10;0.005116 0.20;0.004345 0.30;0.003883 0.40;0.003423 0.50;0.003346 0.60;0.003322 0.70;0.00332 0.80;0.003289 0.90;0.002811 1]  InternalRulePriority=Speed  RndMeth=Simplest
      settings: InputPortMap=u0,u1
  2-D Lookup Table3 : Lookup_n-D  BreakpointsForDimension1=[0 0.10 0.20 0.30 0.40 0.50 0.60 0.70 0.8 0.9 1]  BreakpointsForDimension2=[293.15 313.15]  Table=[2287.7 11897;6122 24515;18460 42098;20975 44453;15254 33098;10440 24492;13903 32975;16694 40007;15784 35937;12165 26430;9118 24795]  InternalRulePriority=Speed  RndMeth=Simplest
      settings: InputPortMap=u0,u1
  Em : Outport
  R0 : Outport  Port=2
  R1 : Outport  Port=3
  C1 : Outport  Port=4
  wires:
  Battery temp/1 -> 2-D Lookup Table3/2, 2-D Lookup Table2/2, 2-D Lookup Table1/2, 2-D Lookup Table/2
  2-D Lookup Table3/1 -> C1/1
  2-D Lookup Table/1 -> Em/1
  SOC/1 -> 2-D Lookup Table3/1, 2-D Lookup Table2/1, 2-D Lookup Table1/1, 2-D Lookup Table/1
  2-D Lookup Table2/1 -> R1/1
  2-D Lookup Table1/1 -> R0/1

== system EV_assigment2/series/Subsystem25/Subsystem1 ==
  Battery Current : Inport
  InitCap(Ah) : Inport  Port=2
  Temp(K) : Inport  Port=3
  Capacity : Lookup_n-D  NumberOfTableDimensions=1  BreakpointsForDimension1=[283.15 313.15]  Table=[28 28]  InternalRulePriority=Speed  RndMeth=Simplest
  Charge accumilator : Integrator  InitialConditionSource=external  UpperSaturationLimit=1  LowerSaturationLimit=0
  Convert to Ah : Gain  Gain=-1/3600
  Divide : Product  Inputs=*/
  LoadAh : Outport
  SOC : Outport  Port=2
  wires:
  Charge accumilator/1 -> Divide/1, LoadAh/1
  Divide/1 -> SOC/1
  Temp(K)/1 -> Capacity/1
  Capacity/1 -> Divide/2
  Battery Current/1 -> Convert to Ah/1
  Convert to Ah/1 -> Charge accumilator/1
  InitCap(Ah)/1 -> Charge accumilator/2

== system EV_assigment2/series/Subsystem26/Subsystem ==
  SOC : Inport
  Battery temp : Inport  Port=2
  2-D Lookup Table : Lookup_n-D  BreakpointsForDimension1=[0 0.10 0.20 0.30 0.40 0.50 0.60 0.70 0.80 0.90 1]  BreakpointsForDimension2=[293.15 313.15]  Table=[3.50 3.51;3.56 3.56; 3.60 3.62;3.64 3.66;3.67 3.69;3.71 3.72;3.79 3.81;3.88 3.89;3.97 3.99;4.08 4.08;4.19 4.19]  InternalRulePriority=Speed  RndMeth=Simplest
      settings: InputPortMap=u0,u1
  2-D Lookup Table1 : Lookup_n-D  BreakpointsForDimension1=[0 0.10 0.20 0.30 0.40 0.50 0.60 0.70 0.80 0.90 1]  BreakpointsForDimension2=[293.15 313.15]  Table=[0.011448 0.009001;0.011038 0.008966;0.011281 0.009126;0.011236 0.00911;0.010959 0.008957;0.010714 0.008797;0.010698 0.008913;0.010712 0.009052;0.010917 0.009044;0.011304 0.008899;0.01160 0.008902]  InternalRulePriority=Speed  RndMeth=Simplest
      settings: InputPortMap=u0,u1
  2-D Lookup Table2 : Lookup_n-D  BreakpointsForDimension1=[0 0.10 0.20 0.30 0.40 0.50 0.60 0.70 0.80 0.90 1]  BreakpointsForDimension2=[293.15 313.15]  Table=[0.010342 0;0.006732 0.10;0.005116 0.20;0.004345 0.30;0.003883 0.40;0.003423 0.50;0.003346 0.60;0.003322 0.70;0.00332 0.80;0.003289 0.90;0.002811 1]  InternalRulePriority=Speed  RndMeth=Simplest
      settings: InputPortMap=u0,u1
  2-D Lookup Table3 : Lookup_n-D  BreakpointsForDimension1=[0 0.10 0.20 0.30 0.40 0.50 0.60 0.70 0.8 0.9 1]  BreakpointsForDimension2=[293.15 313.15]  Table=[2287.7 11897;6122 24515;18460 42098;20975 44453;15254 33098;10440 24492;13903 32975;16694 40007;15784 35937;12165 26430;9118 24795]  InternalRulePriority=Speed  RndMeth=Simplest
      settings: InputPortMap=u0,u1
  Em : Outport
  R0 : Outport  Port=2
  R1 : Outport  Port=3
  C1 : Outport  Port=4
  wires:
  Battery temp/1 -> 2-D Lookup Table3/2, 2-D Lookup Table2/2, 2-D Lookup Table1/2, 2-D Lookup Table/2
  2-D Lookup Table3/1 -> C1/1
  2-D Lookup Table/1 -> Em/1
  SOC/1 -> 2-D Lookup Table3/1, 2-D Lookup Table2/1, 2-D Lookup Table1/1, 2-D Lookup Table/1
  2-D Lookup Table2/1 -> R1/1
  2-D Lookup Table1/1 -> R0/1

== system EV_assigment2/series/Subsystem26/Subsystem1 ==
  Battery Current : Inport
  InitCap(Ah) : Inport  Port=2
  Temp(K) : Inport  Port=3
  Capacity : Lookup_n-D  NumberOfTableDimensions=1  BreakpointsForDimension1=[283.15 313.15]  Table=[28 28]  InternalRulePriority=Speed  RndMeth=Simplest
  Charge accumilator : Integrator  InitialConditionSource=external  UpperSaturationLimit=1  LowerSaturationLimit=0
  Convert to Ah : Gain  Gain=-1/3600
  Divide : Product  Inputs=*/
  LoadAh : Outport
  SOC : Outport  Port=2
  wires:
  Charge accumilator/1 -> Divide/1, LoadAh/1
  Divide/1 -> SOC/1
  Temp(K)/1 -> Capacity/1
  Capacity/1 -> Divide/2
  Battery Current/1 -> Convert to Ah/1
  Convert to Ah/1 -> Charge accumilator/1
  InitCap(Ah)/1 -> Charge accumilator/2

== system EV_assigment2/series/Subsystem27/Subsystem ==
  SOC : Inport
  Battery temp : Inport  Port=2
  2-D Lookup Table : Lookup_n-D  BreakpointsForDimension1=[0 0.10 0.20 0.30 0.40 0.50 0.60 0.70 0.80 0.90 1]  BreakpointsForDimension2=[293.15 313.15]  Table=[3.50 3.51;3.56 3.56; 3.60 3.62;3.64 3.66;3.67 3.69;3.71 3.72;3.79 3.81;3.88 3.89;3.97 3.99;4.08 4.08;4.19 4.19]  InternalRulePriority=Speed  RndMeth=Simplest
      settings: InputPortMap=u0,u1
  2-D Lookup Table1 : Lookup_n-D  BreakpointsForDimension1=[0 0.10 0.20 0.30 0.40 0.50 0.60 0.70 0.80 0.90 1]  BreakpointsForDimension2=[293.15 313.15]  Table=[0.011448 0.009001;0.011038 0.008966;0.011281 0.009126;0.011236 0.00911;0.010959 0.008957;0.010714 0.008797;0.010698 0.008913;0.010712 0.009052;0.010917 0.009044;0.011304 0.008899;0.01160 0.008902]  InternalRulePriority=Speed  RndMeth=Simplest
      settings: InputPortMap=u0,u1
  2-D Lookup Table2 : Lookup_n-D  BreakpointsForDimension1=[0 0.10 0.20 0.30 0.40 0.50 0.60 0.70 0.80 0.90 1]  BreakpointsForDimension2=[293.15 313.15]  Table=[0.010342 0;0.006732 0.10;0.005116 0.20;0.004345 0.30;0.003883 0.40;0.003423 0.50;0.003346 0.60;0.003322 0.70;0.00332 0.80;0.003289 0.90;0.002811 1]  InternalRulePriority=Speed  RndMeth=Simplest
      settings: InputPortMap=u0,u1
  2-D Lookup Table3 : Lookup_n-D  BreakpointsForDimension1=[0 0.10 0.20 0.30 0.40 0.50 0.60 0.70 0.8 0.9 1]  BreakpointsForDimension2=[293.15 313.15]  Table=[2287.7 11897;6122 24515;18460 42098;20975 44453;15254 33098;10440 24492;13903 32975;16694 40007;15784 35937;12165 26430;9118 24795]  InternalRulePriority=Speed  RndMeth=Simplest
      settings: InputPortMap=u0,u1
  Em : Outport
  R0 : Outport  Port=2
  R1 : Outport  Port=3
  C1 : Outport  Port=4
  wires:
  Battery temp/1 -> 2-D Lookup Table3/2, 2-D Lookup Table2/2, 2-D Lookup Table1/2, 2-D Lookup Table/2
  2-D Lookup Table3/1 -> C1/1
  2-D Lookup Table/1 -> Em/1
  SOC/1 -> 2-D Lookup Table3/1, 2-D Lookup Table2/1, 2-D Lookup Table1/1, 2-D Lookup Table/1
  2-D Lookup Table2/1 -> R1/1
  2-D Lookup Table1/1 -> R0/1

== system EV_assigment2/series/Subsystem27/Subsystem1 ==
  Battery Current : Inport
  InitCap(Ah) : Inport  Port=2
  Temp(K) : Inport  Port=3
  Capacity : Lookup_n-D  NumberOfTableDimensions=1  BreakpointsForDimension1=[283.15 313.15]  Table=[28 28]  InternalRulePriority=Speed  RndMeth=Simplest
  Charge accumilator : Integrator  InitialConditionSource=external  UpperSaturationLimit=1  LowerSaturationLimit=0
  Convert to Ah : Gain  Gain=-1/3600
  Divide : Product  Inputs=*/
  LoadAh : Outport
  SOC : Outport  Port=2
  wires:
  Charge accumilator/1 -> Divide/1, LoadAh/1
  Divide/1 -> SOC/1
  Temp(K)/1 -> Capacity/1
  Capacity/1 -> Divide/2
  Battery Current/1 -> Convert to Ah/1
  Convert to Ah/1 -> Charge accumilator/1
  InitCap(Ah)/1 -> Charge accumilator/2

== system EV_assigment2/series/Subsystem28/Subsystem ==
  SOC : Inport
  Battery temp : Inport  Port=2
  2-D Lookup Table : Lookup_n-D  BreakpointsForDimension1=[0 0.10 0.20 0.30 0.40 0.50 0.60 0.70 0.80 0.90 1]  BreakpointsForDimension2=[293.15 313.15]  Table=[3.50 3.51;3.56 3.56; 3.60 3.62;3.64 3.66;3.67 3.69;3.71 3.72;3.79 3.81;3.88 3.89;3.97 3.99;4.08 4.08;4.19 4.19]  InternalRulePriority=Speed  RndMeth=Simplest
      settings: InputPortMap=u0,u1
  2-D Lookup Table1 : Lookup_n-D  BreakpointsForDimension1=[0 0.10 0.20 0.30 0.40 0.50 0.60 0.70 0.80 0.90 1]  BreakpointsForDimension2=[293.15 313.15]  Table=[0.011448 0.009001;0.011038 0.008966;0.011281 0.009126;0.011236 0.00911;0.010959 0.008957;0.010714 0.008797;0.010698 0.008913;0.010712 0.009052;0.010917 0.009044;0.011304 0.008899;0.01160 0.008902]  InternalRulePriority=Speed  RndMeth=Simplest
      settings: InputPortMap=u0,u1
  2-D Lookup Table2 : Lookup_n-D  BreakpointsForDimension1=[0 0.10 0.20 0.30 0.40 0.50 0.60 0.70 0.80 0.90 1]  BreakpointsForDimension2=[293.15 313.15]  Table=[0.010342 0;0.006732 0.10;0.005116 0.20;0.004345 0.30;0.003883 0.40;0.003423 0.50;0.003346 0.60;0.003322 0.70;0.00332 0.80;0.003289 0.90;0.002811 1]  InternalRulePriority=Speed  RndMeth=Simplest
      settings: InputPortMap=u0,u1
  2-D Lookup Table3 : Lookup_n-D  BreakpointsForDimension1=[0 0.10 0.20 0.30 0.40 0.50 0.60 0.70 0.8 0.9 1]  BreakpointsForDimension2=[293.15 313.15]  Table=[2287.7 11897;6122 24515;18460 42098;20975 44453;15254 33098;10440 24492;13903 32975;16694 40007;15784 35937;12165 26430;9118 24795]  InternalRulePriority=Speed  RndMeth=Simplest
      settings: InputPortMap=u0,u1
  Em : Outport
  R0 : Outport  Port=2
  R1 : Outport  Port=3
  C1 : Outport  Port=4
  wires:
  Battery temp/1 -> 2-D Lookup Table3/2, 2-D Lookup Table2/2, 2-D Lookup Table1/2, 2-D Lookup Table/2
  2-D Lookup Table3/1 -> C1/1
  2-D Lookup Table/1 -> Em/1
  SOC/1 -> 2-D Lookup Table3/1, 2-D Lookup Table2/1, 2-D Lookup Table1/1, 2-D Lookup Table/1
  2-D Lookup Table2/1 -> R1/1
  2-D Lookup Table1/1 -> R0/1

== system EV_assigment2/series/Subsystem28/Subsystem1 ==
  Battery Current : Inport
  InitCap(Ah) : Inport  Port=2
  Temp(K) : Inport  Port=3
  Capacity : Lookup_n-D  NumberOfTableDimensions=1  BreakpointsForDimension1=[283.15 313.15]  Table=[28 28]  InternalRulePriority=Speed  RndMeth=Simplest
  Charge accumilator : Integrator  InitialConditionSource=external  UpperSaturationLimit=1  LowerSaturationLimit=0
  Convert to Ah : Gain  Gain=-1/3600
  Divide : Product  Inputs=*/
  LoadAh : Outport
  SOC : Outport  Port=2
  wires:
  Charge accumilator/1 -> Divide/1, LoadAh/1
  Divide/1 -> SOC/1
  Temp(K)/1 -> Capacity/1
  Capacity/1 -> Divide/2
  Battery Current/1 -> Convert to Ah/1
  Convert to Ah/1 -> Charge accumilator/1
  InitCap(Ah)/1 -> Charge accumilator/2

== system EV_assigment2/series/Subsystem3/Subsystem ==
  SOC : Inport
  Battery temp : Inport  Port=2
  2-D Lookup Table : Lookup_n-D  BreakpointsForDimension1=[0 0.10 0.20 0.30 0.40 0.50 0.60 0.70 0.80 0.90 1]  BreakpointsForDimension2=[293.15 313.15]  Table=[3.50 3.51;3.56 3.56; 3.60 3.62;3.64 3.66;3.67 3.69;3.71 3.72;3.79 3.81;3.88 3.89;3.97 3.99;4.08 4.08;4.19 4.19]  InternalRulePriority=Speed  RndMeth=Simplest
      settings: InputPortMap=u0,u1
  2-D Lookup Table1 : Lookup_n-D  BreakpointsForDimension1=[0 0.10 0.20 0.30 0.40 0.50 0.60 0.70 0.80 0.90 1]  BreakpointsForDimension2=[293.15 313.15]  Table=[0.011448 0.009001;0.011038 0.008966;0.011281 0.009126;0.011236 0.00911;0.010959 0.008957;0.010714 0.008797;0.010698 0.008913;0.010712 0.009052;0.010917 0.009044;0.011304 0.008899;0.01160 0.008902]  InternalRulePriority=Speed  RndMeth=Simplest
      settings: InputPortMap=u0,u1
  2-D Lookup Table2 : Lookup_n-D  BreakpointsForDimension1=[0 0.10 0.20 0.30 0.40 0.50 0.60 0.70 0.80 0.90 1]  BreakpointsForDimension2=[293.15 313.15]  Table=[0.010342 0;0.006732 0.10;0.005116 0.20;0.004345 0.30;0.003883 0.40;0.003423 0.50;0.003346 0.60;0.003322 0.70;0.00332 0.80;0.003289 0.90;0.002811 1]  InternalRulePriority=Speed  RndMeth=Simplest
      settings: InputPortMap=u0,u1
  2-D Lookup Table3 : Lookup_n-D  BreakpointsForDimension1=[0 0.10 0.20 0.30 0.40 0.50 0.60 0.70 0.8 0.9 1]  BreakpointsForDimension2=[293.15 313.15]  Table=[2287.7 11897;6122 24515;18460 42098;20975 44453;15254 33098;10440 24492;13903 32975;16694 40007;15784 35937;12165 26430;9118 24795]  InternalRulePriority=Speed  RndMeth=Simplest
      settings: InputPortMap=u0,u1
  Em : Outport
  R0 : Outport  Port=2
  R1 : Outport  Port=3
  C1 : Outport  Port=4
  wires:
  Battery temp/1 -> 2-D Lookup Table3/2, 2-D Lookup Table2/2, 2-D Lookup Table1/2, 2-D Lookup Table/2
  2-D Lookup Table3/1 -> C1/1
  2-D Lookup Table/1 -> Em/1
  SOC/1 -> 2-D Lookup Table3/1, 2-D Lookup Table2/1, 2-D Lookup Table1/1, 2-D Lookup Table/1
  2-D Lookup Table2/1 -> R1/1
  2-D Lookup Table1/1 -> R0/1

== system EV_assigment2/series/Subsystem3/Subsystem1 ==
  Battery Current : Inport
  InitCap(Ah) : Inport  Port=2
  Temp(K) : Inport  Port=3
  Capacity : Lookup_n-D  NumberOfTableDimensions=1  BreakpointsForDimension1=[283.15 313.15]  Table=[28 28]  InternalRulePriority=Speed  RndMeth=Simplest
  Charge accumilator : Integrator  InitialConditionSource=external  UpperSaturationLimit=1  LowerSaturationLimit=0
  Convert to Ah : Gain  Gain=-1/3600
  Divide : Product  Inputs=*/
  LoadAh : Outport
  SOC : Outport  Port=2
  wires:
  Charge accumilator/1 -> Divide/1, LoadAh/1
  Divide/1 -> SOC/1
  Temp(K)/1 -> Capacity/1
  Capacity/1 -> Divide/2
  Battery Current/1 -> Convert to Ah/1
  Convert to Ah/1 -> Charge accumilator/1
  InitCap(Ah)/1 -> Charge accumilator/2

== system EV_assigment2/series/Subsystem4/Subsystem ==
  SOC : Inport
  Battery temp : Inport  Port=2
  2-D Lookup Table : Lookup_n-D  BreakpointsForDimension1=[0 0.10 0.20 0.30 0.40 0.50 0.60 0.70 0.80 0.90 1]  BreakpointsForDimension2=[293.15 313.15]  Table=[3.50 3.51;3.56 3.56; 3.60 3.62;3.64 3.66;3.67 3.69;3.71 3.72;3.79 3.81;3.88 3.89;3.97 3.99;4.08 4.08;4.19 4.19]  InternalRulePriority=Speed  RndMeth=Simplest
      settings: InputPortMap=u0,u1
  2-D Lookup Table1 : Lookup_n-D  BreakpointsForDimension1=[0 0.10 0.20 0.30 0.40 0.50 0.60 0.70 0.80 0.90 1]  BreakpointsForDimension2=[293.15 313.15]  Table=[0.011448 0.009001;0.011038 0.008966;0.011281 0.009126;0.011236 0.00911;0.010959 0.008957;0.010714 0.008797;0.010698 0.008913;0.010712 0.009052;0.010917 0.009044;0.011304 0.008899;0.01160 0.008902]  InternalRulePriority=Speed  RndMeth=Simplest
      settings: InputPortMap=u0,u1
  2-D Lookup Table2 : Lookup_n-D  BreakpointsForDimension1=[0 0.10 0.20 0.30 0.40 0.50 0.60 0.70 0.80 0.90 1]  BreakpointsForDimension2=[293.15 313.15]  Table=[0.010342 0;0.006732 0.10;0.005116 0.20;0.004345 0.30;0.003883 0.40;0.003423 0.50;0.003346 0.60;0.003322 0.70;0.00332 0.80;0.003289 0.90;0.002811 1]  InternalRulePriority=Speed  RndMeth=Simplest
      settings: InputPortMap=u0,u1
  2-D Lookup Table3 : Lookup_n-D  BreakpointsForDimension1=[0 0.10 0.20 0.30 0.40 0.50 0.60 0.70 0.8 0.9 1]  BreakpointsForDimension2=[293.15 313.15]  Table=[2287.7 11897;6122 24515;18460 42098;20975 44453;15254 33098;10440 24492;13903 32975;16694 40007;15784 35937;12165 26430;9118 24795]  InternalRulePriority=Speed  RndMeth=Simplest
      settings: InputPortMap=u0,u1
  Em : Outport
  R0 : Outport  Port=2
  R1 : Outport  Port=3
  C1 : Outport  Port=4
  wires:
  Battery temp/1 -> 2-D Lookup Table3/2, 2-D Lookup Table2/2, 2-D Lookup Table1/2, 2-D Lookup Table/2
  2-D Lookup Table3/1 -> C1/1
  2-D Lookup Table/1 -> Em/1
  SOC/1 -> 2-D Lookup Table3/1, 2-D Lookup Table2/1, 2-D Lookup Table1/1, 2-D Lookup Table/1
  2-D Lookup Table2/1 -> R1/1
  2-D Lookup Table1/1 -> R0/1

== system EV_assigment2/series/Subsystem4/Subsystem1 ==
  Battery Current : Inport
  InitCap(Ah) : Inport  Port=2
  Temp(K) : Inport  Port=3
  Capacity : Lookup_n-D  NumberOfTableDimensions=1  BreakpointsForDimension1=[283.15 313.15]  Table=[28 28]  InternalRulePriority=Speed  RndMeth=Simplest
  Charge accumilator : Integrator  InitialConditionSource=external  UpperSaturationLimit=1  LowerSaturationLimit=0
  Convert to Ah : Gain  Gain=-1/3600
  Divide : Product  Inputs=*/
  LoadAh : Outport
  SOC : Outport  Port=2
  wires:
  Charge accumilator/1 -> Divide/1, LoadAh/1
  Divide/1 -> SOC/1
  Temp(K)/1 -> Capacity/1
  Capacity/1 -> Divide/2
  Battery Current/1 -> Convert to Ah/1
  Convert to Ah/1 -> Charge accumilator/1
  InitCap(Ah)/1 -> Charge accumilator/2
